simulink model "statcom_model_Type2"  (R2023b)
settings: Solver=VariableStepAuto  StartTime=0.0  StopTime=10  RelTol=1e-3
values from neighbouring files (symbols this model uses):
  bc = 1.136    [stat.m]
  g = 2.54    [stat.m]
  gp = 1/rp    (= 0.012706480305)    [stat.m]
  iRref = 1    [stat.m]
  k = 2*sqrt(6)/pi    [stat.m]
  kp = 0.69    [stat.m]
  Rs = 0.01    [stat.m]
  Tw = 0.018    [stat.m]
  vD = 0    [stat.m]
  vQ = 1    [stat.m]
  W0 = Wb    (= 376.991118431)    [stat.m]
  Wb = 2*pi*f0    (= 376.991118431)    [stat.m]
  Xs = 0.15    [stat.m]
settings Model: Creator=HP  LastModifiedBy=HP

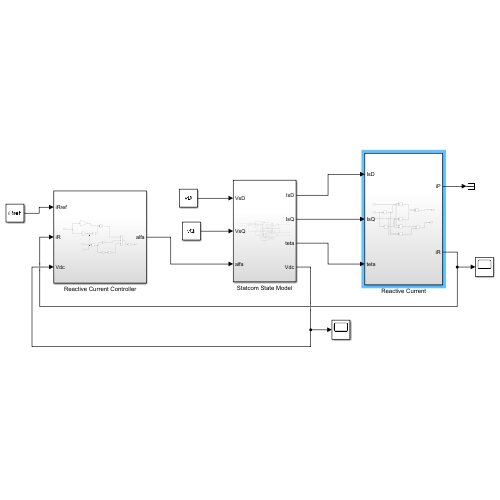
[thumbnail: Simulink's stored preview of the top-level diagram]
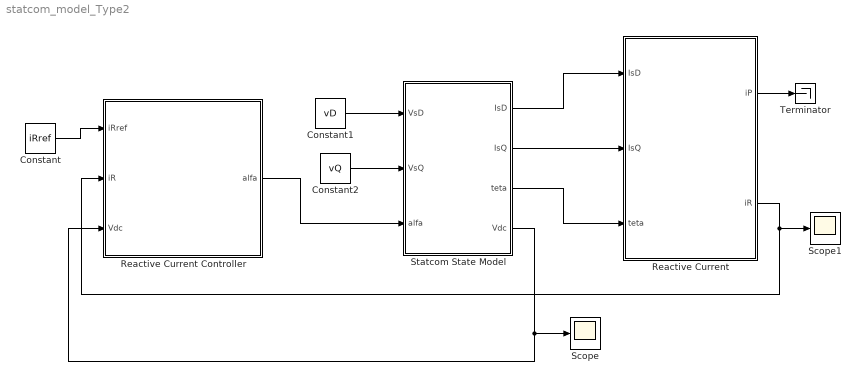
== system statcom_model_Type2 ==
  Constant : Constant  Value=iRref
  Constant1 : Constant  Value=vD
  Constant2 : Constant  Value=vQ
  Reactive Current : Subsystem
  Reactive Current Controller : Subsystem
  Scope : Scope
  Scope1 : Scope
  Statcom State Model : Subsystem
  Terminator : Terminator
  wires:
  Reactive Current Controller/1(alfa) -> Statcom State Model/3(alfa)
  Constant/1 -> Reactive Current Controller/1(iRref)
  Statcom State Model/1(IsD) -> Reactive Current/1(IsD)
  Statcom State Model/2(IsQ) -> Reactive Current/2(IsQ)
  Statcom State Model/3(teta) -> Reactive Current/3(teta)
  Reactive Current/2(iR) -> Reactive Current Controller/2(iR), Scope1/1
  Statcom State Model/4(Vdc) -> Scope/1, Reactive Current Controller/3(Vdc)
  Reactive Current/1(iP) -> Terminator/1
  Constant2/1 -> Statcom State Model/2(VsQ)
  Constant1/1 -> Statcom State Model/1(VsD)

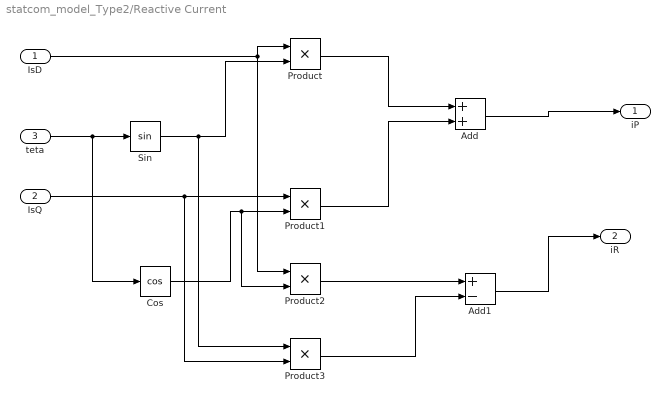
== system statcom_model_Type2/Reactive Current ==
  IsD : Inport
  IsQ : Inport  Port=2
  teta : Inport  Port=3
  Add : Sum
  Add1 : Sum  Inputs=+-
  Cos : Trigonometry  Operator=cos
  Product{,1..3} (4 alike) : Product
  Sin : Trigonometry
  iP : Outport
  iR : Outport  Port=2
  wires:
  Cos/1 -> Product2/2, Product1/2
  teta/1 -> Cos/1, Sin/1
  Sin/1 -> Product3/1, Product/2
  IsQ/1 -> Product3/2, Product1/1
  IsD/1 -> Product/1, Product2/1
  Product/1 -> Add/1
  Product1/1 -> Add/2
  Product3/1 -> Add1/2
  Product2/1 -> Add1/1
  Add/1 -> iP/1
  Add1/1 -> iR/1

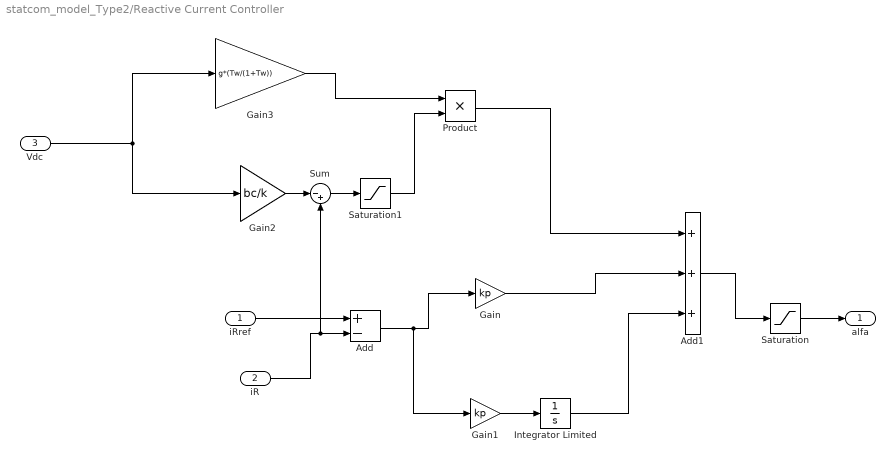
== system statcom_model_Type2/Reactive Current Controller ==
  iRref : Inport
  iR : Inport  Port=2
  Vdc : Inport  Port=3
  Add : Sum  Inputs=+-
  Add1 : Sum  Inputs=+++
  Gain : Gain  Gain=kp
  Gain1 : Gain  Gain=kp
  Gain2 : Gain  Gain=bc/k
  Gain3 : Gain  Gain=g*(Tw/(1+Tw))
  Integrator Limited : Integrator  LimitOutput=on  UpperSaturationLimit=pi/4  LowerSaturationLimit=-pi/4
  Product : Product
  Saturation : Saturate  UpperLimit=pi/4  LowerLimit=-pi/4
  Saturation1 : Saturate
  Sum : Sum  Inputs=|-+
  alfa : Outport
  wires:
  Saturation/1 -> alfa/1
  Add/1 -> Gain1/1, Gain/1
  Add1/1 -> Saturation/1
  Gain/1 -> Add1/2
  Gain3/1 -> Product/1
  Product/1 -> Add1/1
  Gain2/1 -> Sum/1
  Sum/1 -> Saturation1/1
  Saturation1/1 -> Product/2
  Vdc/1 -> Gain2/1, Gain3/1
  Gain1/1 -> Integrator Limited/1
  Integrator Limited/1 -> Add1/3
  iRref/1 -> Add/1
  iR/1 -> Sum/2, Add/2

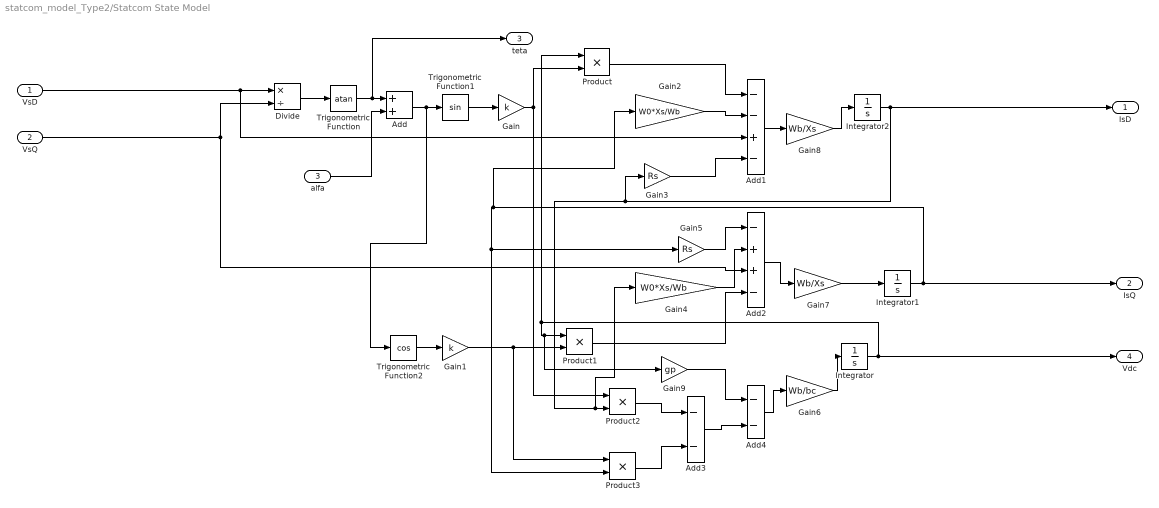
== system statcom_model_Type2/Statcom State Model ==
  VsD : Inport
  VsQ : Inport  Port=2
  alfa : Inport  Port=3
  Add : Sum
  Add1 : Sum  Inputs=--+-
  Add2 : Sum  Inputs=-++-
  Add3 : Sum  Inputs=--
  Add4 : Sum  Inputs=--
  Divide : Product  Inputs=*/
  Gain : Gain  Gain=k
  Gain1 : Gain  Gain=k
  Gain2 : Gain  Gain=W0*Xs/Wb
  Gain3 : Gain  Gain=Rs
  Gain4 : Gain  Gain=W0*Xs/Wb
  Gain5 : Gain  Gain=Rs
  Gain6 : Gain  Gain=Wb/bc
  Gain7 : Gain  Gain=Wb/Xs
  Gain8 : Gain  Gain=Wb/Xs
  Gain9 : Gain  Gain=gp
  Integrator : Integrator
  Integrator1 : Integrator  InitialCondition=1
  Integrator2 : Integrator  InitialCondition=1
  Product{,1..3} (4 alike) : Product
  Trigonometric Function : Trigonometry  Operator=atan
  Trigonometric Function1 : Trigonometry
  Trigonometric Function2 : Trigonometry  Operator=cos
  IsD : Outport
  IsQ : Outport  Port=2
  teta : Outport  Port=3
  Vdc : Outport  Port=4
  wires:
  Gain5/1 -> Add2/1
  VsD/1 -> Add1/3, Divide/1
  Trigonometric Function/1 -> teta/1, Add/1
  Gain/1 -> Product2/1, Product/2
  Integrator1/1 -> IsQ/1, Gain2/1, Gain5/1, Product3/2
  Integrator/1 -> Vdc/1, Product/1, Gain9/1, Product1/1
  Divide/1 -> Trigonometric Function/1
  Gain1/1 -> Product3/1, Product1/2
  Integrator2/1 -> IsD/1, Gain3/1, Gain4/1, Product2/2
  Product3/1 -> Add3/2
  Product2/1 -> Add3/1
  Product1/1 -> Add2/4
  VsQ/1 -> Add2/3, Divide/2
  Gain3/1 -> Add1/4
  Add2/1 -> Gain7/1
  Add4/1 -> Gain6/1
  Add/1 -> Trigonometric Function2/1, Trigonometric Function1/1
  Gain8/1 -> Integrator2/1
  alfa/1 -> Add/2
  Add3/1 -> Add4/2
  Trigonometric Function1/1 -> Gain/1
  Gain9/1 -> Add4/1
  Trigonometric Function2/1 -> Gain1/1
  Gain4/1 -> Add2/2
  Add1/1 -> Gain8/1
  Product/1 -> Add1/1
  Gain7/1 -> Integrator1/1
  Gain2/1 -> Add1/2
  Gain6/1 -> Integrator/1
